simulink model "OrbitSimV1"  (R2021b)
settings: Solver=FixedStepAuto  StartTime=0.0  StopTime=100  FixedStep=.02  RelTol=1e-3
model workspace (MAT data in the model file):
  orbit_altitude = 450000
  r_earth = 6378100
  vel_init = 7640
settings Model: Creator=Ian Lee  LastModifiedBy=Ian Lee

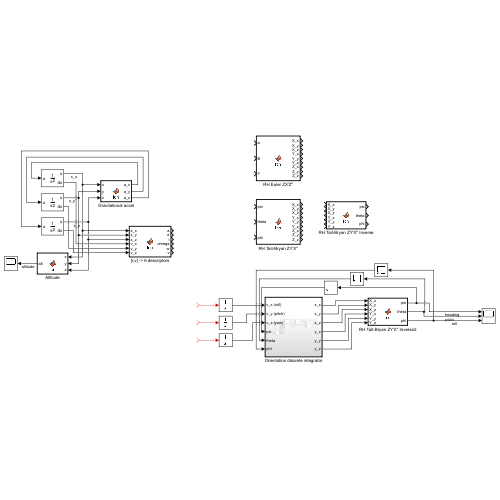
[thumbnail: Simulink's stored preview of the top-level diagram]
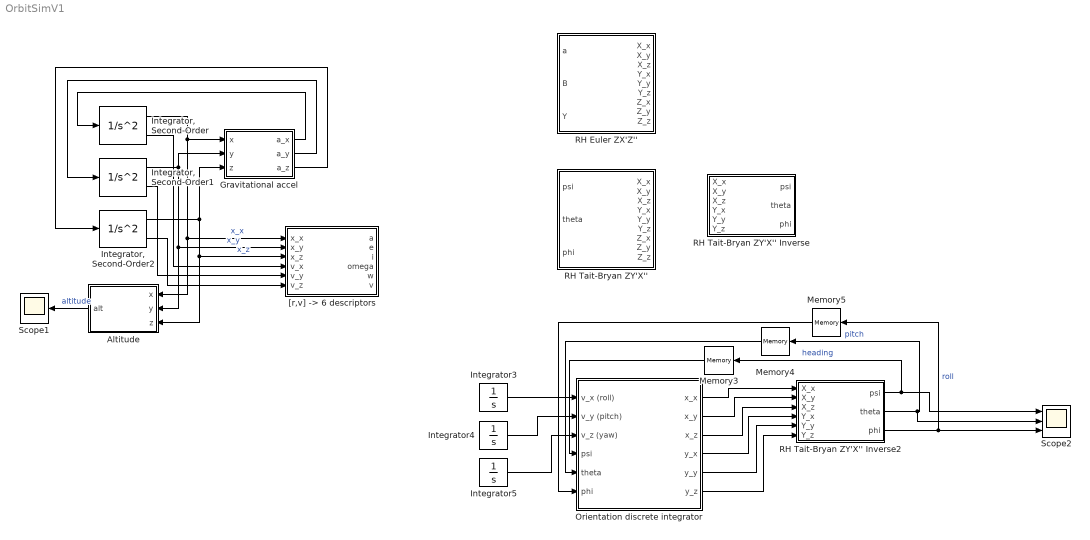
== system OrbitSimV1 ==
  Altitude : MATLAB Function  TreatAsAtomicUnit=on
  Gravitational accel : MATLAB Function  TreatAsAtomicUnit=on
  "Integrator, Second-Order" : SecondOrderIntegrator  ICX=0  ICDXDT=6000
  "Integrator, Second-Order1" : SecondOrderIntegrator  ICX=r_earth + orbit_altitude  ICDXDT=0
  "Integrator, Second-Order2" : SecondOrderIntegrator  ICDXDT=6000
  Integrator3 : Integrator
  Integrator4 : Integrator
  Integrator5 : Integrator
  Memory3 : Memory
  Memory4 : Memory
  Memory5 : Memory
  Orientation discrete integrator : Subsystem  TreatAsAtomicUnit=on
  RH Euler ZX'Z'' : MATLAB Function  TreatAsAtomicUnit=on
  RH Tait-Bryan ZY'X'' : MATLAB Function  TreatAsAtomicUnit=on
  RH Tait-Bryan ZY'X'' Inverse : MATLAB Function  TreatAsAtomicUnit=on
  RH Tait-Bryan ZY'X'' Inverse2 : MATLAB Function  TreatAsAtomicUnit=on
  Scope1 : Scope
  Scope2 : Scope  NumInputPorts=3
  "[r,v] -> 6 descriptors" : MATLAB Function  TreatAsAtomicUnit=on
  wires:
  Gravitational accel/2(a_y) -> "Integrator, Second-Order1"/1
  Gravitational accel/1(a_x) -> "Integrator, Second-Order"/1
  Altitude/1(alt) -> Scope1/1  "altitude"
  "Integrator, Second-Order1"/1 -> "[r,v] -> 6 descriptors"/2(x_y), Altitude/2(y), Gravitational accel/2(y)  "x_y"
  Gravitational accel/3(a_z) -> "Integrator, Second-Order2"/1
  "Integrator, Second-Order2"/1 -> "[r,v] -> 6 descriptors"/3(x_z), Altitude/3(z), Gravitational accel/3(z)  "x_z"
  "Integrator, Second-Order"/1 -> "[r,v] -> 6 descriptors"/1(x_x), Altitude/1(x), Gravitational accel/1(x)  "x_x"
  "Integrator, Second-Order"/2 -> "[r,v] -> 6 descriptors"/4(v_x)
  "Integrator, Second-Order1"/2 -> "[r,v] -> 6 descriptors"/5(v_y)
  "Integrator, Second-Order2"/2 -> "[r,v] -> 6 descriptors"/6(v_z)
  Memory5/1 -> Orientation discrete integrator/6(phi)
  Orientation discrete integrator/1(x_x) -> RH Tait-Bryan ZY'X'' Inverse2/1(X_x)
  RH Tait-Bryan ZY'X'' Inverse2/3(phi) -> Memory5/1, Scope2/3  "roll"
  RH Tait-Bryan ZY'X'' Inverse2/1(psi) -> Scope2/1, Memory3/1  "heading"
  Memory4/1 -> Orientation discrete integrator/5(theta)
  Orientation discrete integrator/4(y_x) -> RH Tait-Bryan ZY'X'' Inverse2/4(Y_x)
  Orientation discrete integrator/6(y_z) -> RH Tait-Bryan ZY'X'' Inverse2/6(Y_z)
  Orientation discrete integrator/2(x_y) -> RH Tait-Bryan ZY'X'' Inverse2/2(X_y)
  Orientation discrete integrator/5(y_y) -> RH Tait-Bryan ZY'X'' Inverse2/5(Y_y)
  Integrator5/1 -> Orientation discrete integrator/3(v_z (yaw))
  Integrator4/1 -> Orientation discrete integrator/2(v_y (pitch))
  Integrator3/1 -> Orientation discrete integrator/1(v_x (roll))
  RH Tait-Bryan ZY'X'' Inverse2/2(theta) -> Scope2/2, Memory4/1  "pitch"
  Orientation discrete integrator/3(x_z) -> RH Tait-Bryan ZY'X'' Inverse2/3(X_z)
  Memory3/1 -> Orientation discrete integrator/4(psi)
  ? -> Integrator3/1
  ? -> Integrator4/1
  ? -> Integrator5/1

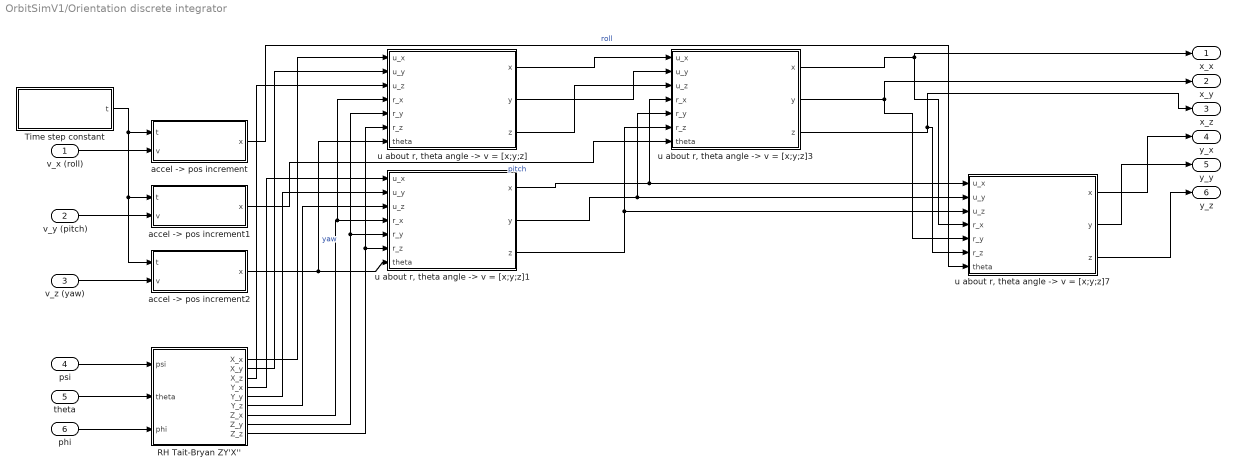
== system OrbitSimV1/Orientation discrete integrator ==
  v_x (roll) : Inport
  v_y (pitch) : Inport  Port=2
  v_z (yaw) : Inport  Port=3
  psi : Inport  Port=4
  theta : Inport  Port=5
  phi : Inport  Port=6
  RH Tait-Bryan ZY'X'' : MATLAB Function  TreatAsAtomicUnit=on
  Time step constant : Subsystem  TreatAsAtomicUnit=on
  "accel -> pos increment" : Subsystem  TreatAsAtomicUnit=on
  "accel -> pos increment1" : Subsystem  TreatAsAtomicUnit=on
  "accel -> pos increment2" : Subsystem  TreatAsAtomicUnit=on
  "u about r, theta angle -> v = [x;y;z]" : Subsystem  TreatAsAtomicUnit=on
  "u about r, theta angle -> v = [x;y;z]1" : Subsystem  TreatAsAtomicUnit=on
  "u about r, theta angle -> v = [x;y;z]3" : Subsystem  TreatAsAtomicUnit=on
  "u about r, theta angle -> v = [x;y;z]7" : Subsystem  TreatAsAtomicUnit=on
  x_x : Outport
  x_y : Outport  Port=2
  x_z : Outport  Port=3
  y_x : Outport  Port=4
  y_y : Outport  Port=5
  y_z : Outport  Port=6
  wires:
  Time step constant/1(t) -> "accel -> pos increment2"/1(t), "accel -> pos increment1"/1(t), "accel -> pos increment"/1(t)
  v_x (roll)/1 -> "accel -> pos increment"/2("v ")
  v_y (pitch)/1 -> "accel -> pos increment1"/2("v ")
  v_z (yaw)/1 -> "accel -> pos increment2"/2("v ")
  "accel -> pos increment1"/1(x) -> "u about r, theta angle -> v = [x;y;z]3"/7(theta)  "pitch"
  "accel -> pos increment2"/1(x) -> "u about r, theta angle -> v = [x;y;z]1"/7(theta), "u about r, theta angle -> v = [x;y;z]"/7(theta)  "yaw"
  psi/1 -> RH Tait-Bryan ZY'X''/1(psi)
  theta/1 -> RH Tait-Bryan ZY'X''/2(theta)
  phi/1 -> RH Tait-Bryan ZY'X''/3(phi)
  RH Tait-Bryan ZY'X''/1(X_x) -> "u about r, theta angle -> v = [x;y;z]"/1(u_x)
  RH Tait-Bryan ZY'X''/2(X_y) -> "u about r, theta angle -> v = [x;y;z]"/2(u_y)
  RH Tait-Bryan ZY'X''/3(X_z) -> "u about r, theta angle -> v = [x;y;z]"/3(u_z)
  RH Tait-Bryan ZY'X''/4(Y_x) -> "u about r, theta angle -> v = [x;y;z]1"/1(u_x)
  RH Tait-Bryan ZY'X''/5(Y_y) -> "u about r, theta angle -> v = [x;y;z]1"/2(u_y)
  RH Tait-Bryan ZY'X''/6(Y_z) -> "u about r, theta angle -> v = [x;y;z]1"/3(u_z)
  "accel -> pos increment"/1(x) -> "u about r, theta angle -> v = [x;y;z]7"/7(theta)  "roll"
  "u about r, theta angle -> v = [x;y;z]"/1(x) -> "u about r, theta angle -> v = [x;y;z]3"/1(u_x)
  "u about r, theta angle -> v = [x;y;z]"/2(y) -> "u about r, theta angle -> v = [x;y;z]3"/2(u_y)
  "u about r, theta angle -> v = [x;y;z]"/3(z) -> "u about r, theta angle -> v = [x;y;z]3"/3(u_z)
  RH Tait-Bryan ZY'X''/7(Z_x) -> "u about r, theta angle -> v = [x;y;z]"/4(r_x), "u about r, theta angle -> v = [x;y;z]1"/4(r_x)
  RH Tait-Bryan ZY'X''/8(Z_y) -> "u about r, theta angle -> v = [x;y;z]"/5(r_y), "u about r, theta angle -> v = [x;y;z]1"/5(r_y)
  RH Tait-Bryan ZY'X''/9(Z_z) -> "u about r, theta angle -> v = [x;y;z]"/6(r_z), "u about r, theta angle -> v = [x;y;z]1"/6(r_z)
  "u about r, theta angle -> v = [x;y;z]1"/1(x) -> "u about r, theta angle -> v = [x;y;z]7"/1(u_x), "u about r, theta angle -> v = [x;y;z]3"/4(r_x)
  "u about r, theta angle -> v = [x;y;z]1"/2(y) -> "u about r, theta angle -> v = [x;y;z]7"/2(u_y), "u about r, theta angle -> v = [x;y;z]3"/5(r_y)
  "u about r, theta angle -> v = [x;y;z]1"/3(z) -> "u about r, theta angle -> v = [x;y;z]7"/3(u_z), "u about r, theta angle -> v = [x;y;z]3"/6(r_z)
  "u about r, theta angle -> v = [x;y;z]3"/1(x) -> x_x/1, "u about r, theta angle -> v = [x;y;z]7"/4(r_x)
  "u about r, theta angle -> v = [x;y;z]3"/2(y) -> x_y/1, "u about r, theta angle -> v = [x;y;z]7"/5(r_y)
  "u about r, theta angle -> v = [x;y;z]3"/3(z) -> x_z/1, "u about r, theta angle -> v = [x;y;z]7"/6(r_z)
  "u about r, theta angle -> v = [x;y;z]7"/1(x) -> y_x/1
  "u about r, theta angle -> v = [x;y;z]7"/2(y) -> y_y/1
  "u about r, theta angle -> v = [x;y;z]7"/3(z) -> y_z/1

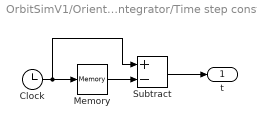
== system OrbitSimV1/Orientation discrete integrator/Time step constant ==
  Clock : Clock
  Memory : Memory  InitialCondition=0.1
  Subtract : Sum  Inputs=+-
  t : Outport
  wires:
  Clock/1 -> Memory/1, Subtract/1
  Memory/1 -> Subtract/2
  Subtract/1 -> t/1

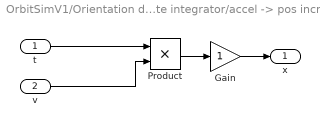
== system OrbitSimV1/Orientation discrete integrator/accel -> pos increment ==
  t : Inport
  "v " : Inport  Port=2
  Gain : Gain
  Product : Product
  x : Outport
  wires:
  t/1 -> Product/1
  "v "/1 -> Product/2
  Product/1 -> Gain/1
  Gain/1 -> x/1

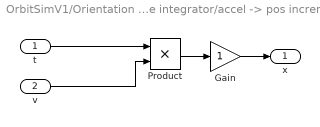
== system OrbitSimV1/Orientation discrete integrator/accel -> pos increment1 ==
  t : Inport
  "v " : Inport  Port=2
  Gain : Gain
  Product : Product
  x : Outport
  wires:
  t/1 -> Product/1
  "v "/1 -> Product/2
  Product/1 -> Gain/1
  Gain/1 -> x/1

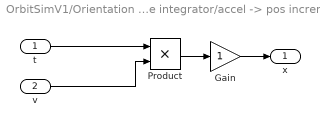
== system OrbitSimV1/Orientation discrete integrator/accel -> pos increment2 ==
  t : Inport
  "v " : Inport  Port=2
  Gain : Gain
  Product : Product
  x : Outport
  wires:
  t/1 -> Product/1
  "v "/1 -> Product/2
  Product/1 -> Gain/1
  Gain/1 -> x/1

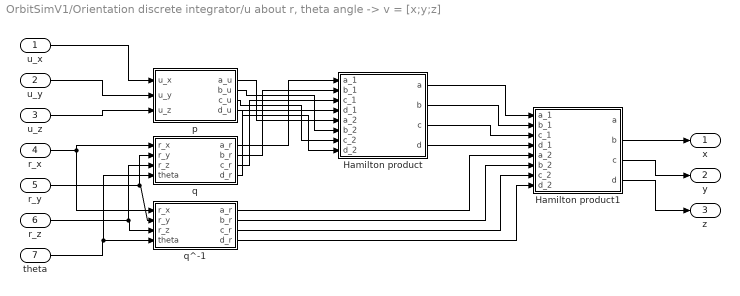
== system OrbitSimV1/Orientation discrete integrator/u about r, theta angle -> v = [x;y;z] ==
  u_x : Inport
  u_y : Inport  Port=2
  u_z : Inport  Port=3
  r_x : Inport  Port=4
  r_y : Inport  Port=5
  r_z : Inport  Port=6
  theta : Inport  Port=7
  Hamilton product : MATLAB Function  TreatAsAtomicUnit=on
  Hamilton product1 : MATLAB Function  TreatAsAtomicUnit=on
  p : MATLAB Function  TreatAsAtomicUnit=on
  q : MATLAB Function  TreatAsAtomicUnit=on
  q^-1 : MATLAB Function  TreatAsAtomicUnit=on
  x : Outport
  y : Outport  Port=2
  z : Outport  Port=3
  wires:
  Hamilton product/1(a) -> Hamilton product1/1(a_1)
  Hamilton product/2(b) -> Hamilton product1/2(b_1)
  Hamilton product/3(c) -> Hamilton product1/3(c_1)
  Hamilton product/4(d) -> Hamilton product1/4(d_1)
  q^-1/1(a_r) -> Hamilton product1/5(a_2)
  q^-1/2(b_r) -> Hamilton product1/6(b_2)
  q^-1/3(c_r) -> Hamilton product1/7(c_2)
  q^-1/4(d_r) -> Hamilton product1/8(d_2)
  theta/1 -> q/4(theta), q^-1/4(theta)
  r_z/1 -> q/3(r_z), q^-1/3(r_z)
  r_y/1 -> q/2(r_y), q^-1/2(r_y)
  r_x/1 -> q/1(r_x), q^-1/1(r_x)
  u_z/1 -> p/3(u_z)
  u_y/1 -> p/2(u_y)
  u_x/1 -> p/1(u_x)
  Hamilton product1/2(b) -> x/1
  Hamilton product1/3(c) -> y/1
  Hamilton product1/4(d) -> z/1
  q/1(a_r) -> Hamilton product/1(a_1)
  q/2(b_r) -> Hamilton product/2(b_1)
  q/3(c_r) -> Hamilton product/3(c_1)
  q/4(d_r) -> Hamilton product/4(d_1)
  p/2(b_u) -> Hamilton product/6(b_2)
  p/3(c_u) -> Hamilton product/7(c_2)
  p/4(d_u) -> Hamilton product/8(d_2)
  p/1(a_u) -> Hamilton product/5(a_2)

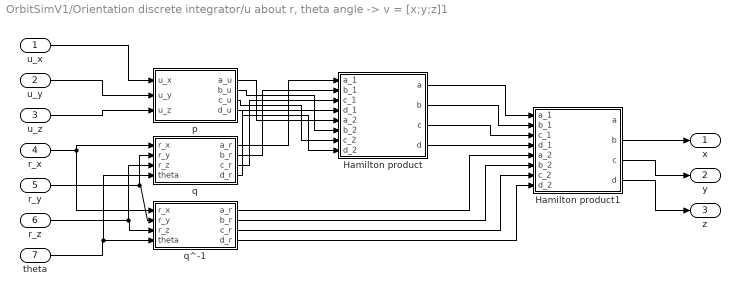
== system OrbitSimV1/Orientation discrete integrator/u about r, theta angle -> v = [x;y;z]1 ==
  u_x : Inport
  u_y : Inport  Port=2
  u_z : Inport  Port=3
  r_x : Inport  Port=4
  r_y : Inport  Port=5
  r_z : Inport  Port=6
  theta : Inport  Port=7
  Hamilton product : MATLAB Function  TreatAsAtomicUnit=on
  Hamilton product1 : MATLAB Function  TreatAsAtomicUnit=on
  p : MATLAB Function  TreatAsAtomicUnit=on
  q : MATLAB Function  TreatAsAtomicUnit=on
  q^-1 : MATLAB Function  TreatAsAtomicUnit=on
  x : Outport
  y : Outport  Port=2
  z : Outport  Port=3
  wires:
  Hamilton product/1(a) -> Hamilton product1/1(a_1)
  Hamilton product/2(b) -> Hamilton product1/2(b_1)
  Hamilton product/3(c) -> Hamilton product1/3(c_1)
  Hamilton product/4(d) -> Hamilton product1/4(d_1)
  q^-1/1(a_r) -> Hamilton product1/5(a_2)
  q^-1/2(b_r) -> Hamilton product1/6(b_2)
  q^-1/3(c_r) -> Hamilton product1/7(c_2)
  q^-1/4(d_r) -> Hamilton product1/8(d_2)
  theta/1 -> q/4(theta), q^-1/4(theta)
  r_z/1 -> q/3(r_z), q^-1/3(r_z)
  r_y/1 -> q/2(r_y), q^-1/2(r_y)
  r_x/1 -> q/1(r_x), q^-1/1(r_x)
  u_z/1 -> p/3(u_z)
  u_y/1 -> p/2(u_y)
  u_x/1 -> p/1(u_x)
  Hamilton product1/2(b) -> x/1
  Hamilton product1/3(c) -> y/1
  Hamilton product1/4(d) -> z/1
  q/1(a_r) -> Hamilton product/1(a_1)
  q/2(b_r) -> Hamilton product/2(b_1)
  q/3(c_r) -> Hamilton product/3(c_1)
  q/4(d_r) -> Hamilton product/4(d_1)
  p/2(b_u) -> Hamilton product/6(b_2)
  p/3(c_u) -> Hamilton product/7(c_2)
  p/4(d_u) -> Hamilton product/8(d_2)
  p/1(a_u) -> Hamilton product/5(a_2)

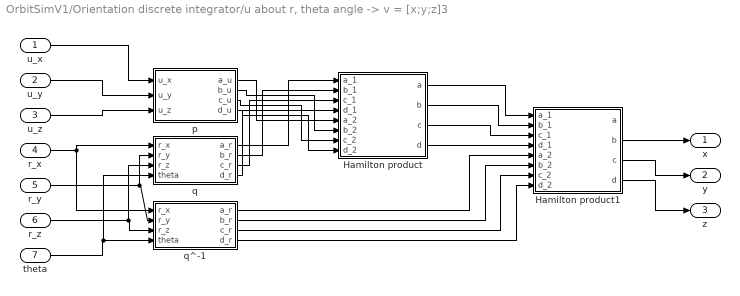
== system OrbitSimV1/Orientation discrete integrator/u about r, theta angle -> v = [x;y;z]3 ==
  u_x : Inport
  u_y : Inport  Port=2
  u_z : Inport  Port=3
  r_x : Inport  Port=4
  r_y : Inport  Port=5
  r_z : Inport  Port=6
  theta : Inport  Port=7
  Hamilton product : MATLAB Function  TreatAsAtomicUnit=on
  Hamilton product1 : MATLAB Function  TreatAsAtomicUnit=on
  p : MATLAB Function  TreatAsAtomicUnit=on
  q : MATLAB Function  TreatAsAtomicUnit=on
  q^-1 : MATLAB Function  TreatAsAtomicUnit=on
  x : Outport
  y : Outport  Port=2
  z : Outport  Port=3
  wires:
  Hamilton product/1(a) -> Hamilton product1/1(a_1)
  Hamilton product/2(b) -> Hamilton product1/2(b_1)
  Hamilton product/3(c) -> Hamilton product1/3(c_1)
  Hamilton product/4(d) -> Hamilton product1/4(d_1)
  q^-1/1(a_r) -> Hamilton product1/5(a_2)
  q^-1/2(b_r) -> Hamilton product1/6(b_2)
  q^-1/3(c_r) -> Hamilton product1/7(c_2)
  q^-1/4(d_r) -> Hamilton product1/8(d_2)
  theta/1 -> q/4(theta), q^-1/4(theta)
  r_z/1 -> q/3(r_z), q^-1/3(r_z)
  r_y/1 -> q/2(r_y), q^-1/2(r_y)
  r_x/1 -> q/1(r_x), q^-1/1(r_x)
  u_z/1 -> p/3(u_z)
  u_y/1 -> p/2(u_y)
  u_x/1 -> p/1(u_x)
  Hamilton product1/2(b) -> x/1
  Hamilton product1/3(c) -> y/1
  Hamilton product1/4(d) -> z/1
  q/1(a_r) -> Hamilton product/1(a_1)
  q/2(b_r) -> Hamilton product/2(b_1)
  q/3(c_r) -> Hamilton product/3(c_1)
  q/4(d_r) -> Hamilton product/4(d_1)
  p/2(b_u) -> Hamilton product/6(b_2)
  p/3(c_u) -> Hamilton product/7(c_2)
  p/4(d_u) -> Hamilton product/8(d_2)
  p/1(a_u) -> Hamilton product/5(a_2)

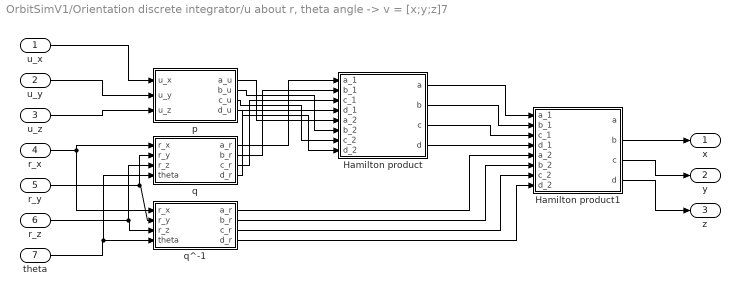
== system OrbitSimV1/Orientation discrete integrator/u about r, theta angle -> v = [x;y;z]7 ==
  u_x : Inport
  u_y : Inport  Port=2
  u_z : Inport  Port=3
  r_x : Inport  Port=4
  r_y : Inport  Port=5
  r_z : Inport  Port=6
  theta : Inport  Port=7
  Hamilton product : MATLAB Function  TreatAsAtomicUnit=on
  Hamilton product1 : MATLAB Function  TreatAsAtomicUnit=on
  p : MATLAB Function  TreatAsAtomicUnit=on
  q : MATLAB Function  TreatAsAtomicUnit=on
  q^-1 : MATLAB Function  TreatAsAtomicUnit=on
  x : Outport
  y : Outport  Port=2
  z : Outport  Port=3
  wires:
  Hamilton product/1(a) -> Hamilton product1/1(a_1)
  Hamilton product/2(b) -> Hamilton product1/2(b_1)
  Hamilton product/3(c) -> Hamilton product1/3(c_1)
  Hamilton product/4(d) -> Hamilton product1/4(d_1)
  q^-1/1(a_r) -> Hamilton product1/5(a_2)
  q^-1/2(b_r) -> Hamilton product1/6(b_2)
  q^-1/3(c_r) -> Hamilton product1/7(c_2)
  q^-1/4(d_r) -> Hamilton product1/8(d_2)
  theta/1 -> q/4(theta), q^-1/4(theta)
  r_z/1 -> q/3(r_z), q^-1/3(r_z)
  r_y/1 -> q/2(r_y), q^-1/2(r_y)
  r_x/1 -> q/1(r_x), q^-1/1(r_x)
  u_z/1 -> p/3(u_z)
  u_y/1 -> p/2(u_y)
  u_x/1 -> p/1(u_x)
  Hamilton product1/2(b) -> x/1
  Hamilton product1/3(c) -> y/1
  Hamilton product1/4(d) -> z/1
  q/1(a_r) -> Hamilton product/1(a_1)
  q/2(b_r) -> Hamilton product/2(b_1)
  q/3(c_r) -> Hamilton product/3(c_1)
  q/4(d_r) -> Hamilton product/4(d_1)
  p/2(b_u) -> Hamilton product/6(b_2)
  p/3(c_u) -> Hamilton product/7(c_2)
  p/4(d_u) -> Hamilton product/8(d_2)
  p/1(a_u) -> Hamilton product/5(a_2)

== matlab function OrbitSimV1/RH Tait-Bryan ZY'X'' Inverse2 ==
  data: X_x input; psi output; X_y input; X_z input; Y_x input; Y_y input; theta output; phi output; Y_z input
function [psi, theta, phi] = fcn(X_x, X_y, X_z, Y_x, Y_y, Y_z)

% psi = heading
% theta = pitch
% phi = bank

psi = atan2(X_y,X_x);
theta = atan2(X_z,sqrt(X_y^2 + X_x^2));
if(-Y_x * sin(psi) + Y_y * cos(psi) > 1)
    n = 1;
elseif(-Y_x * sin(psi) + Y_y * cos(psi) < -1)
    n = -1;
else
    n = -Y_x * sin(psi) + Y_y * cos(psi);
end
if(Y_z > 0)
    phi = acos(n);
else
    phi = -acos(n);
end

== matlab function OrbitSimV1/Orientation discrete integrator/RH Tait-Bryan ZY'X'' ==
  data: psi input; X_x output; theta input; phi input; X_y output; X_z output; Y_x output; Y_y output; Y_z output; Z_x output; Z_y output; Z_z output
function [X_x, X_y, X_z, Y_x, Y_y, Y_z ,Z_x, Z_y, Z_z] = fcn(psi, theta, phi)

% psi = heading
% theta = pitch
% phi = bank

theta = -theta;
final = [
cos(psi) * cos(theta), cos(psi) * sin(theta) * sin(phi) - cos(phi) * sin(psi), sin(psi) * sin(phi) + cos(psi) * cos(phi) * sin(theta);
cos(theta) * sin(psi), cos(psi) * cos(phi) + sin(psi) * sin(theta) * sin(phi), cos(phi) * sin(psi) * sin(theta) - cos(psi) * sin(phi);
-sin(theta), cos(theta) * sin(phi), cos(theta) * cos(phi);
];

X1 = [1;0;0];
Y1 = [0;1;0];
Z1 = [0;0;1];

X2 = final * X1;
Y2 = final * Y1;
Z2 = final * Z1;

X_x = X2(1);
X_y = X2(2);
X_z = X2(3);
Y_x = Y2(1);
Y_y = Y2(2);
Y_z = Y2(3);
Z_x = Z2(1);
Z_y = Z2(2);
Z_z = Z2(3);

== matlab function OrbitSimV1/Orientation discrete integrator/u about r, theta angle -> v = [x;y;z]/Hamilton product ==
  data: a_1 input; a output; b_1 input; c_1 input; d_1 input; a_2 input; b_2 input; c_2 input; d_2 input; b output; c output; d output
function [a, b, c, d] = fcn(a_1, b_1, c_1, d_1, a_2, b_2, c_2, d_2)

a = a_1 * a_2 - b_1 * b_2 - c_1 * c_2 - d_1 * d_2;
b = a_1 * b_2 + b_1 * a_2 + c_1 * d_2 - d_1 * c_2;
c = a_1 * c_2 - b_1 * d_2 + c_1 * a_2 + d_1 * b_2;
d = a_1 * d_2 + b_1 * c_2 - c_1 * b_2 + d_1 * a_2;

== matlab function OrbitSimV1/Orientation discrete integrator/u about r, theta angle -> v = [x;y;z]/Hamilton product1 ==
  data: a_1 input; a output; b_1 input; c_1 input; d_1 input; a_2 input; b_2 input; c_2 input; d_2 input; b output; c output; d output
function [a, b, c, d] = fcn(a_1, b_1, c_1, d_1, a_2, b_2, c_2, d_2)

a = a_1 * a_2 - b_1 * b_2 - c_1 * c_2 - d_1 * d_2;
b = a_1 * b_2 + b_1 * a_2 + c_1 * d_2 - d_1 * c_2;
c = a_1 * c_2 - b_1 * d_2 + c_1 * a_2 + d_1 * b_2;
d = a_1 * d_2 + b_1 * c_2 - c_1 * b_2 + d_1 * a_2;

== matlab function OrbitSimV1/Orientation discrete integrator/u about r, theta angle -> v = [x;y;z]/p ==
  data: u_x input; u_y input; u_z input; a_u output; b_u output; c_u output; d_u output
function [a_u, b_u, c_u, d_u] = fcn(u_x, u_y, u_z)
a_u = 0;
b_u = u_x;
c_u = u_y;
d_u = u_z;

== matlab function OrbitSimV1/Orientation discrete integrator/u about r, theta angle -> v = [x;y;z]/q ==
  data: r_x input; a_r output; r_y input; r_z input; theta input; b_r output; c_r output; d_r output
function [a_r, b_r, c_r, d_r] = fcn(r_x, r_y, r_z, theta)

a_r = cos(theta / 2);
b_r = r_x * sin(theta / 2);
c_r = r_y * sin(theta / 2);
d_r = r_z * sin(theta / 2);

== matlab function OrbitSimV1/Orientation discrete integrator/u about r, theta angle -> v = [x;y;z]/q^-1 ==
  data: r_x input; a_r output; r_y input; r_z input; theta input; b_r output; c_r output; d_r output
function [a_r, b_r, c_r, d_r] = fcn(r_x, r_y, r_z, theta)

a_r = cos(theta / 2);
b_r = r_x * -sin(theta / 2);
c_r = r_y * -sin(theta / 2);
d_r = r_z * -sin(theta / 2);

== matlab function OrbitSimV1/Orientation discrete integrator/u about r, theta angle -> v = [x;y;z]1/Hamilton product ==
  data: a_1 input; a output; b_1 input; c_1 input; d_1 input; a_2 input; b_2 input; c_2 input; d_2 input; b output; c output; d output
function [a, b, c, d] = fcn(a_1, b_1, c_1, d_1, a_2, b_2, c_2, d_2)

a = a_1 * a_2 - b_1 * b_2 - c_1 * c_2 - d_1 * d_2;
b = a_1 * b_2 + b_1 * a_2 + c_1 * d_2 - d_1 * c_2;
c = a_1 * c_2 - b_1 * d_2 + c_1 * a_2 + d_1 * b_2;
d = a_1 * d_2 + b_1 * c_2 - c_1 * b_2 + d_1 * a_2;

== matlab function OrbitSimV1/Gravitational accel ==
  data: x input; a_x output; y input; z input; a_y output; a_z output
function [a_x, a_y, a_z] = fcn(x, y, z)
% determine acceleration
d = sqrt(x^2 + y^2 + z^2);
a = -((6.67408*10^-11) * (5.97219*10^24)) / d^2;
% x,y,z unit vector for direction
x1 = x / d;
y1 = y / d;
z1 = z / d;
% x,y,z acceleration vectors
a_x = a * x1;
a_y = a * y1;
a_z = a * z1;

== matlab function OrbitSimV1/Orientation discrete integrator/u about r, theta angle -> v = [x;y;z]1/Hamilton product1 ==
  data: a_1 input; a output; b_1 input; c_1 input; d_1 input; a_2 input; b_2 input; c_2 input; d_2 input; b output; c output; d output
function [a, b, c, d] = fcn(a_1, b_1, c_1, d_1, a_2, b_2, c_2, d_2)

a = a_1 * a_2 - b_1 * b_2 - c_1 * c_2 - d_1 * d_2;
b = a_1 * b_2 + b_1 * a_2 + c_1 * d_2 - d_1 * c_2;
c = a_1 * c_2 - b_1 * d_2 + c_1 * a_2 + d_1 * b_2;
d = a_1 * d_2 + b_1 * c_2 - c_1 * b_2 + d_1 * a_2;

== matlab function OrbitSimV1/Orientation discrete integrator/u about r, theta angle -> v = [x;y;z]1/p ==
  data: u_x input; u_y input; u_z input; a_u output; b_u output; c_u output; d_u output
function [a_u, b_u, c_u, d_u] = fcn(u_x, u_y, u_z)
a_u = 0;
b_u = u_x;
c_u = u_y;
d_u = u_z;

== matlab function OrbitSimV1/Orientation discrete integrator/u about r, theta angle -> v = [x;y;z]1/q ==
  data: r_x input; a_r output; r_y input; r_z input; theta input; b_r output; c_r output; d_r output
function [a_r, b_r, c_r, d_r] = fcn(r_x, r_y, r_z, theta)

a_r = cos(theta / 2);
b_r = r_x * sin(theta / 2);
c_r = r_y * sin(theta / 2);
d_r = r_z * sin(theta / 2);

== matlab function OrbitSimV1/Orientation discrete integrator/u about r, theta angle -> v = [x;y;z]1/q^-1 ==
  data: r_x input; a_r output; r_y input; r_z input; theta input; b_r output; c_r output; d_r output
function [a_r, b_r, c_r, d_r] = fcn(r_x, r_y, r_z, theta)

a_r = cos(theta / 2);
b_r = r_x * -sin(theta / 2);
c_r = r_y * -sin(theta / 2);
d_r = r_z * -sin(theta / 2);

== matlab function OrbitSimV1/Orientation discrete integrator/u about r, theta angle -> v = [x;y;z]3/Hamilton product ==
  data: a_1 input; a output; b_1 input; c_1 input; d_1 input; a_2 input; b_2 input; c_2 input; d_2 input; b output; c output; d output
function [a, b, c, d] = fcn(a_1, b_1, c_1, d_1, a_2, b_2, c_2, d_2)

a = a_1 * a_2 - b_1 * b_2 - c_1 * c_2 - d_1 * d_2;
b = a_1 * b_2 + b_1 * a_2 + c_1 * d_2 - d_1 * c_2;
c = a_1 * c_2 - b_1 * d_2 + c_1 * a_2 + d_1 * b_2;
d = a_1 * d_2 + b_1 * c_2 - c_1 * b_2 + d_1 * a_2;

== matlab function OrbitSimV1/Orientation discrete integrator/u about r, theta angle -> v = [x;y;z]3/Hamilton product1 ==
  data: a_1 input; a output; b_1 input; c_1 input; d_1 input; a_2 input; b_2 input; c_2 input; d_2 input; b output; c output; d output
function [a, b, c, d] = fcn(a_1, b_1, c_1, d_1, a_2, b_2, c_2, d_2)

a = a_1 * a_2 - b_1 * b_2 - c_1 * c_2 - d_1 * d_2;
b = a_1 * b_2 + b_1 * a_2 + c_1 * d_2 - d_1 * c_2;
c = a_1 * c_2 - b_1 * d_2 + c_1 * a_2 + d_1 * b_2;
d = a_1 * d_2 + b_1 * c_2 - c_1 * b_2 + d_1 * a_2;

== matlab function OrbitSimV1/Orientation discrete integrator/u about r, theta angle -> v = [x;y;z]3/p ==
  data: u_x input; u_y input; u_z input; a_u output; b_u output; c_u output; d_u output
function [a_u, b_u, c_u, d_u] = fcn(u_x, u_y, u_z)
a_u = 0;
b_u = u_x;
c_u = u_y;
d_u = u_z;

== matlab function OrbitSimV1/Orientation discrete integrator/u about r, theta angle -> v = [x;y;z]3/q ==
  data: r_x input; a_r output; r_y input; r_z input; theta input; b_r output; c_r output; d_r output
function [a_r, b_r, c_r, d_r] = fcn(r_x, r_y, r_z, theta)

a_r = cos(theta / 2);
b_r = r_x * sin(theta / 2);
c_r = r_y * sin(theta / 2);
d_r = r_z * sin(theta / 2);

== matlab function OrbitSimV1/[r,v] -> 6 descriptors ==
  data: x_x input; a output; x_y input; x_z input; v_x input; v_y input; v_z input; e output; i output; omega output; w output; v output
function [a, e, i, omega, w, v] = fcn(x_x, x_y, x_z, v_x, v_y, v_z)

% by math magic, we know (SEE RESEARCH FILES\Orbital mechanics.pdf):
% e is the eccentricity vector, that points from apoapsis to periapsis with
% magnitude = orbit's scalar eccentricity; mu is standard gravitational
% parameter: mu = G(m1 + m2), in this case satellite mass is negligible. 

r = [x_x, x_y, x_z];
r_hat = r / norm(r);
r_dot = [v_x, v_y, v_z];
h = cross(r,r_dot);
mu = 3.986004418*10^14;
ecc_vec = (1 / mu) * (cross(r_dot,h) - mu * r_hat);
e = norm(ecc_vec); % e

i = acos(h(3) / norm(h)); % i

spec_mech_e = ((norm(r_dot))^2 / 2) - mu / norm(r);
a = (-mu) / (2 * spec_mech_e); % a

if(i ~= 0)
    n = cross([0,0,1],h);
    omega = acos(n(1) / norm(n)); % omega
    if(n(2) < 0)
        omega = 2*pi - omega;
    end
    
    w = acos(dot(n,ecc_vec) / (norm(n) * e)); % w
    if(ecc_vec(3) < 0)
        w = 2*pi - w;
    end
    
    v = acos(dot(ecc_vec,r) / (norm(r) * e)); % v
    if(dot(r,r_dot) < 0)
        w = 2*pi - w;
    end
else
    omega = 0;
    w = 0;
    v = 0;
end

== matlab function OrbitSimV1/Orientation discrete integrator/u about r, theta angle -> v = [x;y;z]3/q^-1 ==
  data: r_x input; a_r output; r_y input; r_z input; theta input; b_r output; c_r output; d_r output
function [a_r, b_r, c_r, d_r] = fcn(r_x, r_y, r_z, theta)

a_r = cos(theta / 2);
b_r = r_x * -sin(theta / 2);
c_r = r_y * -sin(theta / 2);
d_r = r_z * -sin(theta / 2);

== matlab function OrbitSimV1/Orientation discrete integrator/u about r, theta angle -> v = [x;y;z]7/Hamilton product ==
  data: a_1 input; a output; b_1 input; c_1 input; d_1 input; a_2 input; b_2 input; c_2 input; d_2 input; b output; c output; d output
function [a, b, c, d] = fcn(a_1, b_1, c_1, d_1, a_2, b_2, c_2, d_2)

a = a_1 * a_2 - b_1 * b_2 - c_1 * c_2 - d_1 * d_2;
b = a_1 * b_2 + b_1 * a_2 + c_1 * d_2 - d_1 * c_2;
c = a_1 * c_2 - b_1 * d_2 + c_1 * a_2 + d_1 * b_2;
d = a_1 * d_2 + b_1 * c_2 - c_1 * b_2 + d_1 * a_2;

== matlab function OrbitSimV1/Orientation discrete integrator/u about r, theta angle -> v = [x;y;z]7/Hamilton product1 ==
  data: a_1 input; a output; b_1 input; c_1 input; d_1 input; a_2 input; b_2 input; c_2 input; d_2 input; b output; c output; d output
function [a, b, c, d] = fcn(a_1, b_1, c_1, d_1, a_2, b_2, c_2, d_2)

a = a_1 * a_2 - b_1 * b_2 - c_1 * c_2 - d_1 * d_2;
b = a_1 * b_2 + b_1 * a_2 + c_1 * d_2 - d_1 * c_2;
c = a_1 * c_2 - b_1 * d_2 + c_1 * a_2 + d_1 * b_2;
d = a_1 * d_2 + b_1 * c_2 - c_1 * b_2 + d_1 * a_2;

== matlab function OrbitSimV1/Orientation discrete integrator/u about r, theta angle -> v = [x;y;z]7/p ==
  data: u_x input; u_y input; u_z input; a_u output; b_u output; c_u output; d_u output
function [a_u, b_u, c_u, d_u] = fcn(u_x, u_y, u_z)
a_u = 0;
b_u = u_x;
c_u = u_y;
d_u = u_z;

== matlab function OrbitSimV1/Orientation discrete integrator/u about r, theta angle -> v = [x;y;z]7/q ==
  data: r_x input; a_r output; r_y input; r_z input; theta input; b_r output; c_r output; d_r output
function [a_r, b_r, c_r, d_r] = fcn(r_x, r_y, r_z, theta)

a_r = cos(theta / 2);
b_r = r_x * sin(theta / 2);
c_r = r_y * sin(theta / 2);
d_r = r_z * sin(theta / 2);

== matlab function OrbitSimV1/Orientation discrete integrator/u about r, theta angle -> v = [x;y;z]7/q^-1 ==
  data: r_x input; a_r output; r_y input; r_z input; theta input; b_r output; c_r output; d_r output
function [a_r, b_r, c_r, d_r] = fcn(r_x, r_y, r_z, theta)

a_r = cos(theta / 2);
b_r = r_x * -sin(theta / 2);
c_r = r_y * -sin(theta / 2);
d_r = r_z * -sin(theta / 2);

== matlab function OrbitSimV1/Altitude ==
  data: x input; alt output; y input; z input
function alt = fcn(x, y, z)

alt = sqrt(x^2 + y^2 + z^2) - (6.3781*10^6);

== matlab function OrbitSimV1/RH Euler ZX'Z'' ==
  data: a input; X_x output; B input; X_y output; X_z output; Y input; Y_x output; Y_y output; Y_z output; Z_x output; Z_y output; Z_z output
function [X_x, X_y, X_z, Y_x, Y_y, Y_z ,Z_x, Z_y, Z_z] = fcn(a, B, Y)
% a = alpha, B = beta, Y = gamma
% (a, B, Y) method (x-convention): a: rotate about Z, B: rotate about X, Y:
% rotate about Z
% Z X Z rotation.

final = [
cos(a) * cos(Y) - cos(B) * sin(a) * sin(Y), -cos(a) * sin(Y) - cos(B) * cos(Y) * sin(a), sin(a) * sin(B);
cos(Y) * sin(a) + cos(a) * cos(B) * sin(Y), cos(a) * cos(B) * cos(Y) - sin(a) * sin(Y), -cos(a) * sin(B);
sin(B) * sin(Y), cos(Y) * sin(B), cos(B);
];

X1 = [1;0;0];
Y1 = [0;1;0];
Z1 = [0;0;1];

X2 = final * X1;
Y2 = final * Y1;
Z2 = final * Z1;

X_x = X2(1);
X_y = X2(2);
X_z = X2(3);
Y_x = Y2(1);
Y_y = Y2(2);
Y_z = Y2(3);
Z_x = Z2(1);
Z_y = Z2(2);
Z_z = Z2(3);

== matlab function OrbitSimV1/RH Tait-Bryan ZY'X'' ==
  data: psi input; X_x output; theta input; phi input; X_y output; X_z output; Y_x output; Y_y output; Y_z output; Z_x output; Z_y output; Z_z output
function [X_x, X_y, X_z, Y_x, Y_y, Y_z ,Z_x, Z_y, Z_z] = fcn(psi, theta, phi)

% psi = heading
% theta = pitch
% phi = bank

theta = -theta;
final = [
cos(psi) * cos(theta), cos(psi) * sin(theta) * sin(phi) - cos(phi) * sin(psi), sin(psi) * sin(phi) + cos(psi) * cos(phi) * sin(theta);
cos(theta) * sin(psi), cos(psi) * cos(phi) + sin(psi) * sin(theta) * sin(phi), cos(phi) * sin(psi) * sin(theta) - cos(psi) * sin(phi);
-sin(theta), cos(theta) * sin(phi), cos(theta) * cos(phi);
];

X1 = [1;0;0];
Y1 = [0;1;0];
Z1 = [0;0;1];

X2 = final * X1;
Y2 = final * Y1;
Z2 = final * Z1;

X_x = X2(1);
X_y = X2(2);
X_z = X2(3);
Y_x = Y2(1);
Y_y = Y2(2);
Y_z = Y2(3);
Z_x = Z2(1);
Z_y = Z2(2);
Z_z = Z2(3);

== matlab function OrbitSimV1/RH Tait-Bryan ZY'X'' Inverse ==
  data: X_x input; psi output; X_y input; X_z input; Y_x input; Y_y input; theta output; phi output; Y_z input
function [psi, theta, phi] = fcn(X_x, X_y, X_z, Y_x, Y_y, Y_z)

% psi = heading
% theta = pitch
% phi = bank

psi = atan2(X_y,X_x);
theta = atan2(X_z,sqrt(X_y^2 + X_x^2));
if(Y_z > 0)
    phi = acos(-Y_x * sin(psi) + Y_y * cos(psi));
else
    phi = -acos(-Y_x * sin(psi) + Y_y * cos(psi));
end
